simulink model "basebot_velocity_turnrate"  (R2025a)
settings: Solver=ode45  StartTime=0.0  StopTime=1.5  RelTol=1e-3
InitFcn:
  | if exist('piDesign.mat','file'), load('piDesign.mat'); end; gear=9.6; wrad=0.0315; B=0.15; limit_9V=9; Ts=0.001;
values from neighbouring files (symbols this model uses):
  den = [4.84323072847e-08 4.8661333765e-05 8.000321026e-05]    [piDesign.mat]    (also in transferFunction.m = conv([L R], [J D]) + [0 0 K^2])
  Kp = 0.2    [piDesign.m]    (also in piDesign.mat)
  num = 0.00868283239801    [piDesign.mat]    (also in transferFunction.m = K)
settings Model: Creator=leon3  LastModifiedBy=leon3

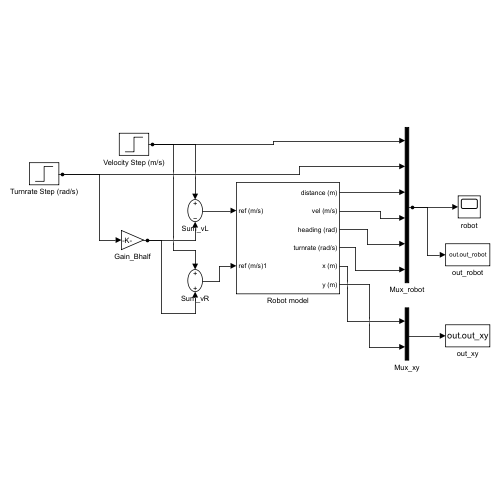
[thumbnail: Simulink's stored preview of the top-level diagram]
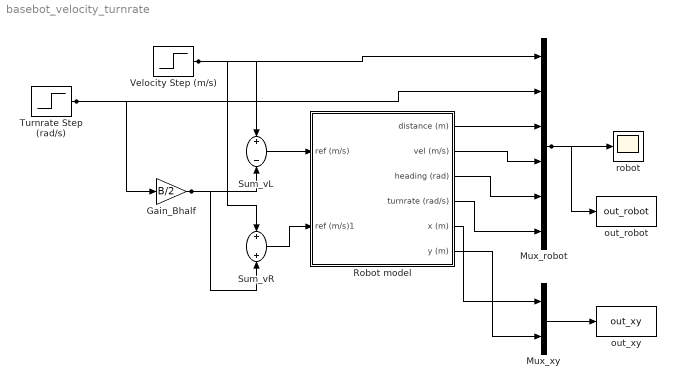
== system basebot_velocity_turnrate ==
  Gain_Bhalf : Gain  Gain=B/2
  Mux_robot : Mux  Inputs=6
  Mux_xy : Mux  Inputs=2
  Robot model : Subsystem
  Sum_vL : Sum  Inputs=+-
  Sum_vR : Sum
  Turnrate Step (rad/s) : Step  Time=0.5  After=1.0  SampleTime=0
  Velocity Step (m/s) : Step  Time=0.1  After=0.6  SampleTime=0
  out_robot : ToWorkspace  VariableName=out_robot  SaveFormat=Timeseries  SampleTime=-1
  out_xy : ToWorkspace  VariableName=out_xy  SaveFormat=Timeseries  SampleTime=-1
  robot : Scope
  wires:
  Gain_Bhalf/1 -> Sum_vR/2, Sum_vL/2
  Sum_vR/1 -> Robot model/2(ref (m/s)1)
  Sum_vL/1 -> Robot model/1(ref (m/s))
  Velocity Step (m/s)/1 -> Sum_vR/1, Mux_robot/1, Sum_vL/1
  Turnrate Step (rad/s)/1 -> Mux_robot/2, Gain_Bhalf/1
  Robot model/3(heading (rad)) -> Mux_robot/5
  Robot model/2(vel (m/s)) -> Mux_robot/4
  Robot model/1(distance (m)) -> Mux_robot/3
  Robot model/4(turnrate (rad/s)) -> Mux_robot/6
  Robot model/5(x (m)) -> Mux_xy/1
  Robot model/6(y (m)) -> Mux_xy/2
  Mux_robot/1 -> robot/1, out_robot/1
  Mux_xy/1 -> out_xy/1

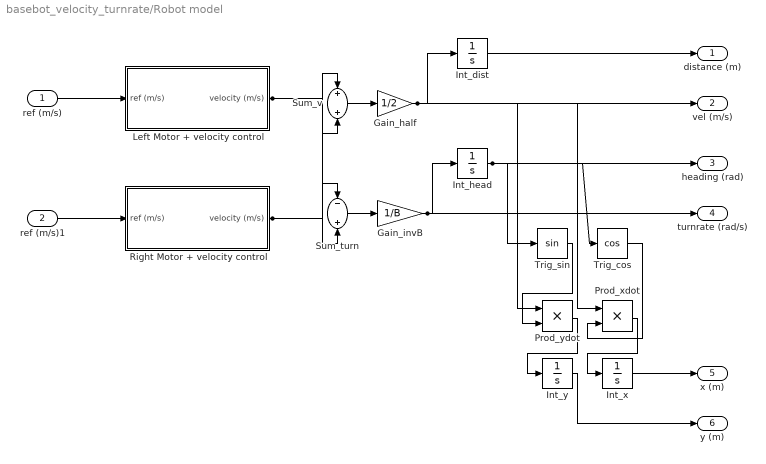
== system basebot_velocity_turnrate/Robot model ==
  ref (m/s) : Inport
  ref (m/s)1 : Inport  Port=2
  Gain_half : Gain  Gain=1/2
  Gain_invB : Gain  Gain=1/B
  Int_dist : Integrator
  Int_head : Integrator
  Int_x : Integrator
  Int_y : Integrator
  Left Motor + velocity control : Subsystem
  Prod_xdot : Product  Inputs=**
  Prod_ydot : Product  Inputs=**
  Right Motor + velocity control : Subsystem
  Sum_turn : Sum  Inputs=-+
  Sum_v : Sum
  Trig_cos : Trigonometry  Operator=cos
  Trig_sin : Trigonometry
  distance (m) : Outport
  vel (m/s) : Outport  Port=2
  heading (rad) : Outport  Port=3
  turnrate (rad/s) : Outport  Port=4
  x (m) : Outport  Port=5
  y (m) : Outport  Port=6
  wires:
  ref (m/s)/1 -> Left Motor + velocity control/1(ref (m/s))
  ref (m/s)1/1 -> Right Motor + velocity control/1(ref (m/s))
  Left Motor + velocity control/1(velocity (m/s)) -> Sum_v/1, Sum_turn/1
  Right Motor + velocity control/1(velocity (m/s)) -> Sum_v/2, Sum_turn/2
  Sum_v/1 -> Gain_half/1
  Sum_turn/1 -> Gain_invB/1
  Gain_half/1 -> Int_dist/1, Prod_xdot/1, Prod_ydot/1, vel (m/s)/1
  Gain_invB/1 -> Int_head/1, turnrate (rad/s)/1
  Int_head/1 -> Trig_sin/1, Trig_cos/1, heading (rad)/1
  Trig_cos/1 -> Prod_xdot/2
  Prod_xdot/1 -> Int_x/1
  Trig_sin/1 -> Prod_ydot/2
  Prod_ydot/1 -> Int_y/1
  Int_dist/1 -> distance (m)/1
  Int_x/1 -> x (m)/1
  Int_y/1 -> y (m)/1

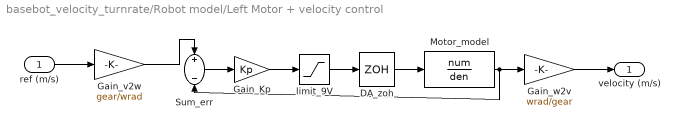
== system basebot_velocity_turnrate/Robot model/Left Motor + velocity control ==
  ref (m/s) : Inport
  DA_zoh : ZeroOrderHold  SampleTime=0.001
  Gain_Kp : Gain  Gain=Kp
  Gain_v2w : Gain  Gain=gear/wrad
  Gain_w2v : Gain  Gain=wrad/gear
  Motor_model : TransferFcn  Numerator=num  Denominator=den
  Sum_err : Sum  Inputs=+-
  limit_9V : Saturate  UpperLimit=9  LowerLimit=-9
  velocity (m/s) : Outport
  wires:
  ref (m/s)/1 -> Gain_v2w/1
  Gain_v2w/1 -> Sum_err/1
  Sum_err/1 -> Gain_Kp/1
  Gain_Kp/1 -> limit_9V/1
  limit_9V/1 -> DA_zoh/1
  DA_zoh/1 -> Motor_model/1
  Motor_model/1 -> Gain_w2v/1, Sum_err/2
  Gain_w2v/1 -> velocity (m/s)/1

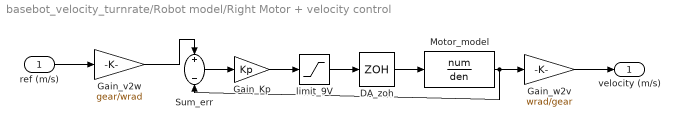
== system basebot_velocity_turnrate/Robot model/Right Motor + velocity control ==
  ref (m/s) : Inport
  DA_zoh : ZeroOrderHold  SampleTime=0.001
  Gain_Kp : Gain  Gain=Kp
  Gain_v2w : Gain  Gain=gear/wrad
  Gain_w2v : Gain  Gain=wrad/gear
  Motor_model : TransferFcn  Numerator=num  Denominator=den
  Sum_err : Sum  Inputs=+-
  limit_9V : Saturate  UpperLimit=9  LowerLimit=-9
  velocity (m/s) : Outport
  wires:
  ref (m/s)/1 -> Gain_v2w/1
  Gain_v2w/1 -> Sum_err/1
  Sum_err/1 -> Gain_Kp/1
  Gain_Kp/1 -> limit_9V/1
  limit_9V/1 -> DA_zoh/1
  DA_zoh/1 -> Motor_model/1
  Motor_model/1 -> Gain_w2v/1, Sum_err/2
  Gain_w2v/1 -> velocity (m/s)/1
